simulink model "flight_controller"  (R2020a)
settings: Solver=FixedStepAuto  StartTime=0.0  StopTime=10  FixedStep=0.01  RelTol=1e-3
InitFcn:
  | flight_controller_setup % Run setup script for this simulation
values from neighbouring files (symbols this model uses):
  ki_dtheta = kp_dtheta*z_c    (= 0.1)    [PID_design_setup.m]
  kp_dtheta = 10^(K_dB/20)    [PID_design_setup.m]
  kp_theta = PID_theta.Kp    [flight_controller_setup.m]
  MM = [-1, 1 ... (first row only)    [flight_controller_payload_setup.m]    (also in flight_controller_setup.m)
  N_dtheta = Inf    (= inf)    [flight_controller_payload_setup.m]    (also in flight_controller_setup.m = 1/Tf_dtheta)
  N_dz = 5*2*pi    (= 31.4159265359)    [flight_controller_payload_setup.m]    (also in flight_controller_setup.m = 1/Tf_dz)
  x0 = zeros(nx,1)    [flight_controller_payload_setup.m]    (also in flight_controller_setup.m = zeros(6,1))
undefined symbols (not defined in the file or in its folder): kd_dtheta, kd_dz, ki_dz, kp_dz, kp_z
libraries: simulink x6
settings Model: Creator=murray  LastModifiedBy=murray

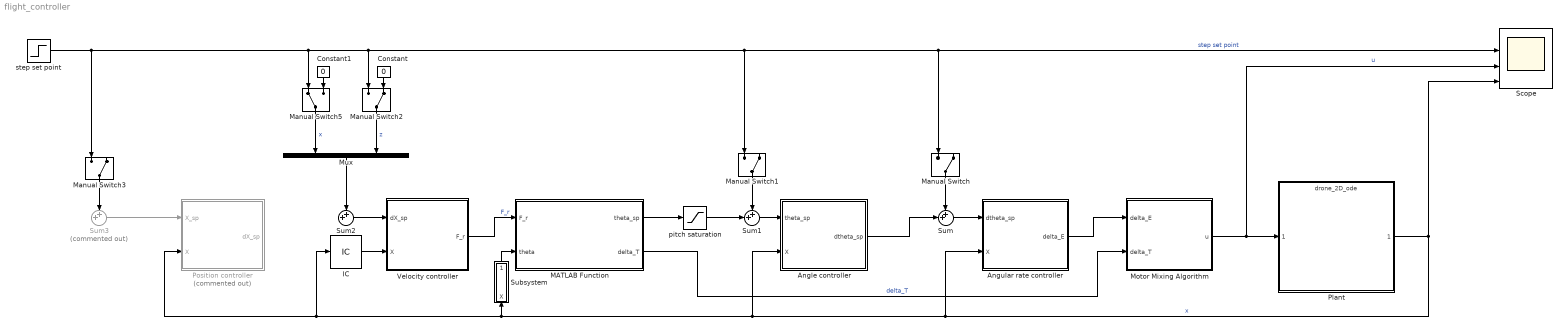
== system flight_controller ==
  Angle controller : Subsystem
  Angular rate controller : Subsystem
  Constant : Constant  Value=0
  Constant1 : Constant  Value=0
  IC : InitialCondition  Value=x0
  MATLAB Function : MATLAB Function  TreatAsAtomicUnit=on
  Manual Switch{,1..3} (4 alike) : ManualSwitch  CurrentSetting=0
  Manual Switch5 : ManualSwitch
  Motor Mixing Algorithm : Subsystem
  Mux : Mux  Inputs=2
  Plant : ModelReference  ModelNameDialog=drone_2D_ode  SimulationMode=Normal  ModelReferenceVersion=1.20
  Position controller : Subsystem  Commented=on
  Scope : Scope  NumInputPorts=4
  Subsystem : Subsystem
  Sum : Sum  Inputs=++|
  Sum1 : Sum  Inputs=++|
  Sum2 : Sum  Inputs=++|
  Sum3 : Sum  Commented=on  Inputs=++|
  Velocity controller : Subsystem
  pitch saturation : Saturate  UpperLimit=pi/2  LowerLimit=-pi/2
  step set point : Step  Time=2  SampleTime=0
  wires:
  Plant/1 -> Angle controller/2(X), IC/1, Position controller/2(X), Subsystem/1(X), Angular rate controller/2(X), Scope/4  "x"
  Angular rate controller/1(delta_E) -> Motor Mixing Algorithm/1(delta_E)
  MATLAB Function/2(delta_T) -> Motor Mixing Algorithm/2(delta_T)  "delta_T"
  Motor Mixing Algorithm/1(u) -> Scope/3, Plant/1  "u"
  Angle controller/1(dtheta_sp) -> Sum/2
  Sum/1 -> Angular rate controller/1(dtheta_sp)
  Manual Switch/1 -> Sum/1
  Manual Switch1/1 -> Sum1/1
  Sum1/1 -> Angle controller/1(theta_sp)
  step set point/1 -> Manual Switch/1, Scope/2, Manual Switch1/1, Manual Switch2/1, Manual Switch5/1, Manual Switch3/1  "step set point"
  Manual Switch3/1 -> Sum3/1
  Sum3/1 -> Position controller/1(X_sp)
  MATLAB Function/1(theta_sp) -> pitch saturation/1
  pitch saturation/1 -> Sum1/2
  Sum2/1 -> Velocity controller/1(dX_sp)
  Velocity controller/1(F_r) -> MATLAB Function/1(F_r)  "F_r"
  Manual Switch5/1 -> Mux/1  "x"
  Mux/1 -> Sum2/1
  IC/1 -> Velocity controller/2(X)
  Constant/1 -> Manual Switch2/2
  Constant1/1 -> Manual Switch5/2
  Manual Switch2/1 -> Mux/2  "z"
  Subsystem/1(theta) -> MATLAB Function/2(theta)

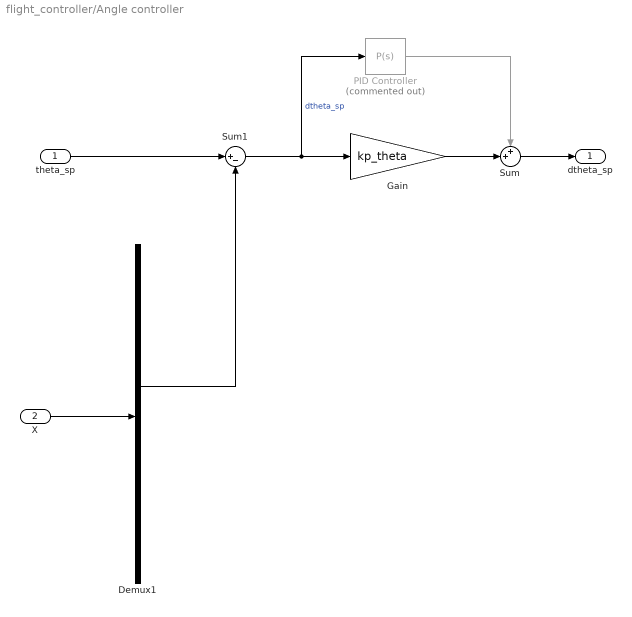
== system flight_controller/Angle controller ==
  theta_sp : Inport
  X : Inport  Port=2
  Demux1 : Demux  Outputs=6
  Gain : Gain  Gain=kp_theta
  PID Controller : simulink/Continuous/PID Controller  Commented=on  Controller=P  Form=Parallel  TimeDomain=Continuous-time  UseExternalTs=off  SampleTime=-1  IntegratorMethod=Forward Euler  FilterMethod=Forward Euler  ControllerParametersSource=internal  P=kp_theta  I=1  D=0  UseFilter=on  N=100  TunerSelectOption=Transfer Function Based (PID Tuner App)  InitialConditionSource=internal  InitialConditionForIntegrator=0  InitialConditionForFilter=0  DifferentiatorICPrevScaledInput=0  ExternalReset=none  TrackingMode=off  Kt=1  LimitOutput=off  UpperSaturationLimit=inf  LowerSaturationLimit=-inf  LinearizeAsGain=on  AntiWindupMode=none  Kb=1  POutMin=[]  POutMax=[]  IOutMin=[]  IOutMax=[]  DOutMin=[]  DOutMax=[]  NOutMin=[]  NOutMax=[]  SumOutMin=[]  SumOutMax=[]  SaturationOutMin=[]  SaturationOutMax=[]  PParamMin=[]  PParamMax=[]  IParamMin=[]  IParamMax=[]  DParamMin=[]  DParamMax=[]  NParamMin=[]  NParamMax=[]  KbParamMin=[]  KbParamMax=[]  KtParamMin=[]  KtParamMax=[]  KbOutMin=[]  KbOutMax=[]  KtOutMin=[]  KtOutMax=[]  IntegratorOutMin=[]  IntegratorOutMax=[]  FilterOutMin=[]  FilterOutMax=[]  SumI1OutMin=[]  SumI1OutMax=[]  SumI2OutMin=[]  SumI2OutMax=[]  SumI3OutMin=[]  SumI3OutMax=[]  SumI4OutMin=[]  SumI4OutMax=[]  SumDOutMin=[]  SumDOutMax=[]  DifferentiatorOutMin=[]  DifferentiatorOutMax=[]  FilterDiffOutCoefMin=[]  FilterDiffOutCoefMax=[]  ReciprocalOutMin=[]  ReciprocalOutMax=[]  SumDenOutMin=[]  SumDenOutMax=[]  SumNumOutMin=[]  SumNumOutMax=[]  DivideOutMin=[]  DivideOutMax=[]  UdiffTsProdOutMin=[]  UdiffTsProdOutMax=[]  NTsProdOutMin=[]  NTsProdOutMax=[]  UintegralTsProdOutMin=[]  UintegralTsProdOutMax=[]  UngainTsProdOutMin=[]  UngainTsProdOutMax=[]  IntegratorContinuousStateAttributes=''  IntegratorStateMustResolveToSignalObject=off  IntegratorRTWStateStorageClass=Auto  FilterContinuousStateAttributes=''  FilterStateMustResolveToSignalObject=off  FilterRTWStateStorageClass=Auto  ParallelPVariant=InternalParameters  IdealPVariant=Disabled  IVariant=Disabled  DVariant=Disabled  IntegratorVariant=Disabled  SatVariant=Disabled  AWVariant=Disabled  PCopyVariant=Disabled  TRVariant=Disabled  FdbkBlocksVariant=Forward  IdealPFdbkVariant=Disabled  SatFdbkVariant=Disabled  DerivativeFilterVariant=Disabled  NVariant=Disabled  NCopyVariant=Disabled_SignalSpec  FilterICVariant=Disabled  IntegratorICVariant=Disabled  ExternalResetVariant=Disabled  TRSumVariant=Passthrough  SumFdbkVariant=Disabled  SumVariant=Passthrough_P  TsampFilterVariant=InternalTs  TsampNgainVariant=Passthrough  TsampIntegralVariant=Disabled_SignalSpec
  Sum : Sum  Inputs=++|
  Sum1 : Sum  Inputs=|+-
  dtheta_sp : Outport
  wires:
  Sum1/1 -> PID Controller/1, Gain/1  "dtheta_sp"
  theta_sp/1 -> Sum1/1
  Sum/1 -> dtheta_sp/1
  PID Controller/1 -> Sum/1
  Gain/1 -> Sum/2
  X/1 -> Demux1/1
  Demux1/3 -> Sum1/2

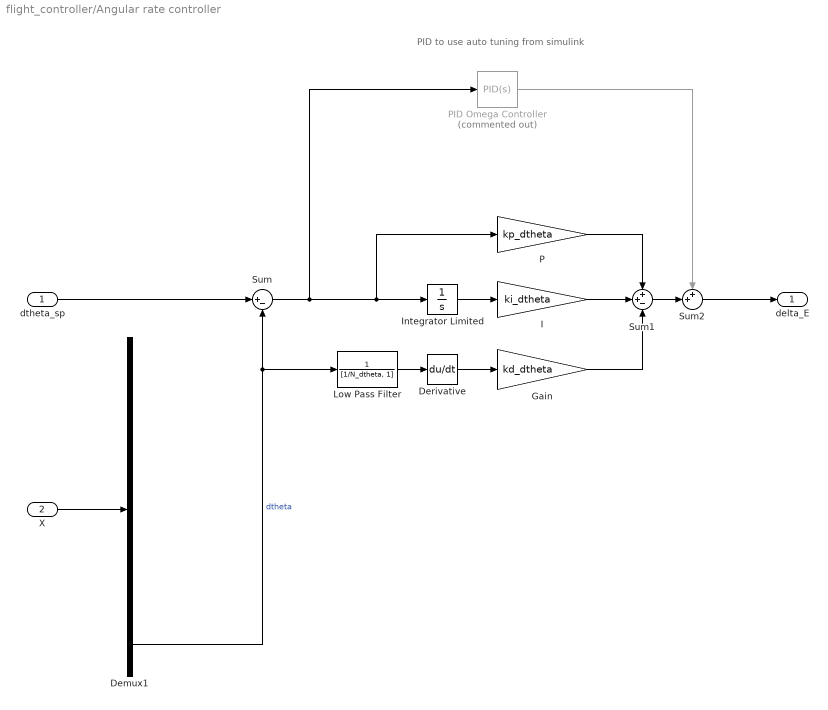
== system flight_controller/Angular rate controller ==
  note: PID to use auto tuning from simulink
  dtheta_sp : Inport
  X : Inport  Port=2
  Demux1 : Demux  Outputs=6
  Derivative : Derivative
  Gain : Gain  Gain=kd_dtheta
  I : Gain  Gain=ki_dtheta
  Integrator Limited : Integrator  LimitOutput=on  UpperSaturationLimit=10  LowerSaturationLimit=-10
  Low Pass Filter : TransferFcn  Denominator=[1/N_dtheta, 1]
  P : Gain  Gain=kp_dtheta
  PID Omega Controller : simulink/Continuous/PID Controller  Commented=on  Controller=PID  Form=Parallel  TimeDomain=Continuous-time  UseExternalTs=off  SampleTime=-1  IntegratorMethod=Forward Euler  FilterMethod=Forward Euler  ControllerParametersSource=internal  P=kp_dtheta  I=ki_dtheta  D=kd_dtheta  UseFilter=on  N=N_dtheta  TunerSelectOption=Transfer Function Based (PID Tuner App)  InitialConditionSource=internal  InitialConditionForIntegrator=0  InitialConditionForFilter=0  DifferentiatorICPrevScaledInput=0  ExternalReset=none  TrackingMode=off  Kt=1  LimitOutput=off  UpperSaturationLimit=inf  LowerSaturationLimit=-inf  LinearizeAsGain=on  AntiWindupMode=none  Kb=1  POutMin=[]  POutMax=[]  IOutMin=[]  IOutMax=[]  DOutMin=[]  DOutMax=[]  NOutMin=[]  NOutMax=[]  SumOutMin=[]  SumOutMax=[]  SaturationOutMin=[]  SaturationOutMax=[]  PParamMin=[]  PParamMax=[]  IParamMin=[]  IParamMax=[]  DParamMin=[]  DParamMax=[]  NParamMin=[]  NParamMax=[]  KbParamMin=[]  KbParamMax=[]  KtParamMin=[]  KtParamMax=[]  KbOutMin=[]  KbOutMax=[]  KtOutMin=[]  KtOutMax=[]  IntegratorOutMin=[]  IntegratorOutMax=[]  FilterOutMin=[]  FilterOutMax=[]  SumI1OutMin=[]  SumI1OutMax=[]  SumI2OutMin=[]  SumI2OutMax=[]  SumI3OutMin=[]  SumI3OutMax=[]  SumI4OutMin=[]  SumI4OutMax=[]  SumDOutMin=[]  SumDOutMax=[]  DifferentiatorOutMin=[]  DifferentiatorOutMax=[]  FilterDiffOutCoefMin=[]  FilterDiffOutCoefMax=[]  ReciprocalOutMin=[]  ReciprocalOutMax=[]  SumDenOutMin=[]  SumDenOutMax=[]  SumNumOutMin=[]  SumNumOutMax=[]  DivideOutMin=[]  DivideOutMax=[]  UdiffTsProdOutMin=[]  UdiffTsProdOutMax=[]  NTsProdOutMin=[]  NTsProdOutMax=[]  UintegralTsProdOutMin=[]  UintegralTsProdOutMax=[]  UngainTsProdOutMin=[]  UngainTsProdOutMax=[]  IntegratorContinuousStateAttributes=''  IntegratorStateMustResolveToSignalObject=off  IntegratorRTWStateStorageClass=Auto  FilterContinuousStateAttributes=''  FilterStateMustResolveToSignalObject=off  FilterRTWStateStorageClass=Auto  ParallelPVariant=InternalParameters  IdealPVariant=Disabled  IVariant=InternalParameters  DVariant=InternalParameters  IntegratorVariant=Continuous  SatVariant=Disabled  AWVariant=Passthrough  PCopyVariant=Disabled  TRVariant=Disabled  FdbkBlocksVariant=Forward  IdealPFdbkVariant=Disabled  SatFdbkVariant=Disabled  DerivativeFilterVariant=ContFilter  NVariant=InternalParameters  NCopyVariant=Disabled  FilterICVariant=InternalICsFilter  IntegratorICVariant=InternalICs  ExternalResetVariant=Disabled  TRSumVariant=Passthrough  SumFdbkVariant=Disabled  SumVariant=Sum_PID  TsampFilterVariant=InternalTs  TsampNgainVariant=Passthrough  TsampIntegralVariant=Passthrough
  Sum : Sum  Inputs=|+-
  Sum1 : Sum  Inputs=++-
  Sum2 : Sum  Inputs=++|
  delta_E : Outport
  wires:
  dtheta_sp/1 -> Sum/1
  Sum/1 -> P/1, Integrator Limited/1, PID Omega Controller/1
  Integrator Limited/1 -> I/1
  Derivative/1 -> Gain/1
  I/1 -> Sum1/2
  P/1 -> Sum1/1
  Gain/1 -> Sum1/3
  Sum1/1 -> Sum2/2
  Sum2/1 -> delta_E/1
  PID Omega Controller/1 -> Sum2/1
  Low Pass Filter/1 -> Derivative/1
  X/1 -> Demux1/1
  Demux1/6 -> Low Pass Filter/1, Sum/2  "dtheta"

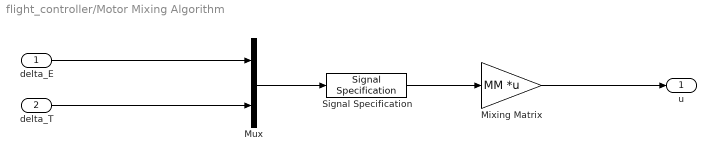
== system flight_controller/Motor Mixing Algorithm ==
  delta_E : Inport
  delta_T : Inport  Port=2
  Mixing Matrix : Gain  Gain=MM  Multiplication=Matrix(K*u)
  Mux : Mux  Inputs=2
  Signal Specification : SignalSpecification  Dimensions=[2, 1]
  u : Outport  LockScale=on
  wires:
  delta_T/1 -> Mux/2
  delta_E/1 -> Mux/1
  Mixing Matrix/1 -> u/1
  Mux/1 -> Signal Specification/1
  Signal Specification/1 -> Mixing Matrix/1

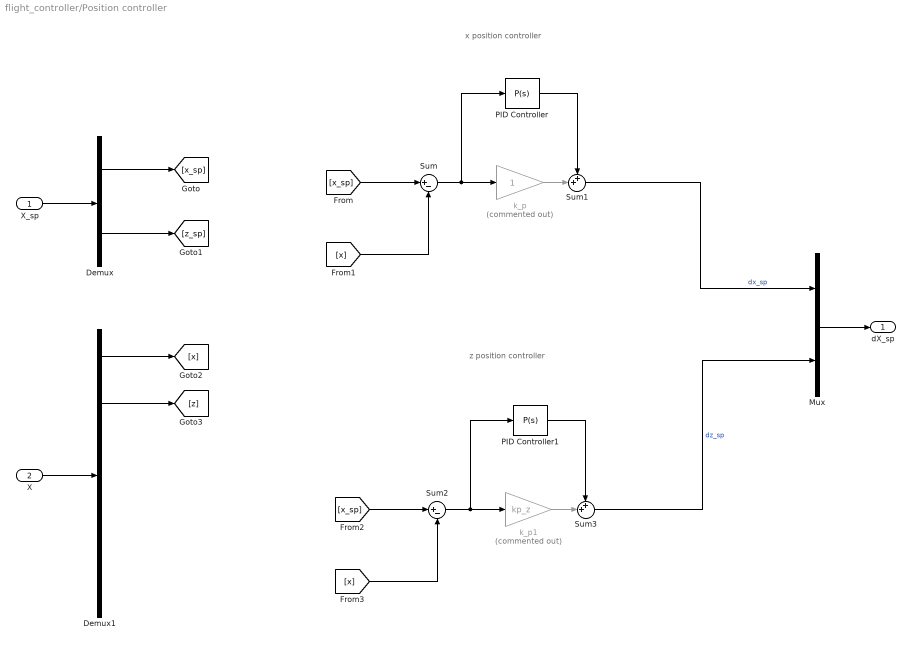
== system flight_controller/Position controller ==
  note: x position controller
  note: z position controller
  X_sp : Inport
  X : Inport  Port=2
  Demux : Demux  Outputs=2
  Demux1 : Demux  Outputs=6
  Mux : Mux  Inputs=2
  PID Controller : simulink/Continuous/PID Controller  Controller=P  Form=Parallel  TimeDomain=Continuous-time  UseExternalTs=off  SampleTime=-1  IntegratorMethod=Forward Euler  FilterMethod=Forward Euler  ControllerParametersSource=internal  P=1  I=1  D=0  UseFilter=on  N=100  TunerSelectOption=Transfer Function Based (PID Tuner App)  InitialConditionSource=internal  InitialConditionForIntegrator=0  InitialConditionForFilter=0  DifferentiatorICPrevScaledInput=0  ExternalReset=none  TrackingMode=off  Kt=1  LimitOutput=off  UpperSaturationLimit=inf  LowerSaturationLimit=-inf  LinearizeAsGain=on  AntiWindupMode=none  Kb=1  POutMin=[]  POutMax=[]  IOutMin=[]  IOutMax=[]  DOutMin=[]  DOutMax=[]  NOutMin=[]  NOutMax=[]  SumOutMin=[]  SumOutMax=[]  SaturationOutMin=[]  SaturationOutMax=[]  PParamMin=[]  PParamMax=[]  IParamMin=[]  IParamMax=[]  DParamMin=[]  DParamMax=[]  NParamMin=[]  NParamMax=[]  KbParamMin=[]  KbParamMax=[]  KtParamMin=[]  KtParamMax=[]  KbOutMin=[]  KbOutMax=[]  KtOutMin=[]  KtOutMax=[]  IntegratorOutMin=[]  IntegratorOutMax=[]  FilterOutMin=[]  FilterOutMax=[]  SumI1OutMin=[]  SumI1OutMax=[]  SumI2OutMin=[]  SumI2OutMax=[]  SumI3OutMin=[]  SumI3OutMax=[]  SumI4OutMin=[]  SumI4OutMax=[]  SumDOutMin=[]  SumDOutMax=[]  DifferentiatorOutMin=[]  DifferentiatorOutMax=[]  FilterDiffOutCoefMin=[]  FilterDiffOutCoefMax=[]  ReciprocalOutMin=[]  ReciprocalOutMax=[]  SumDenOutMin=[]  SumDenOutMax=[]  SumNumOutMin=[]  SumNumOutMax=[]  DivideOutMin=[]  DivideOutMax=[]  UdiffTsProdOutMin=[]  UdiffTsProdOutMax=[]  NTsProdOutMin=[]  NTsProdOutMax=[]  UintegralTsProdOutMin=[]  UintegralTsProdOutMax=[]  UngainTsProdOutMin=[]  UngainTsProdOutMax=[]  IntegratorContinuousStateAttributes=''  IntegratorStateMustResolveToSignalObject=off  IntegratorRTWStateStorageClass=Auto  FilterContinuousStateAttributes=''  FilterStateMustResolveToSignalObject=off  FilterRTWStateStorageClass=Auto  ParallelPVariant=InternalParameters  IdealPVariant=Disabled  IVariant=Disabled  DVariant=Disabled  IntegratorVariant=Disabled  SatVariant=Disabled  AWVariant=Disabled  PCopyVariant=Disabled  TRVariant=Disabled  FdbkBlocksVariant=Forward  IdealPFdbkVariant=Disabled  SatFdbkVariant=Disabled  DerivativeFilterVariant=Disabled  NVariant=Disabled  NCopyVariant=Disabled_SignalSpec  FilterICVariant=Disabled  IntegratorICVariant=Disabled  ExternalResetVariant=Disabled  TRSumVariant=Passthrough  SumFdbkVariant=Disabled  SumVariant=Passthrough_P  TsampFilterVariant=InternalTs  TsampNgainVariant=Passthrough  TsampIntegralVariant=Disabled_SignalSpec
  PID Controller1 : simulink/Continuous/PID Controller  Controller=P  Form=Parallel  TimeDomain=Continuous-time  UseExternalTs=off  SampleTime=-1  IntegratorMethod=Forward Euler  FilterMethod=Forward Euler  ControllerParametersSource=internal  P=kp_z  I=1  D=0  UseFilter=on  N=100  TunerSelectOption=Transfer Function Based (PID Tuner App)  InitialConditionSource=internal  InitialConditionForIntegrator=0  InitialConditionForFilter=0  DifferentiatorICPrevScaledInput=0  ExternalReset=none  TrackingMode=off  Kt=1  LimitOutput=off  UpperSaturationLimit=inf  LowerSaturationLimit=-inf  LinearizeAsGain=on  AntiWindupMode=none  Kb=1  POutMin=[]  POutMax=[]  IOutMin=[]  IOutMax=[]  DOutMin=[]  DOutMax=[]  NOutMin=[]  NOutMax=[]  SumOutMin=[]  SumOutMax=[]  SaturationOutMin=[]  SaturationOutMax=[]  PParamMin=[]  PParamMax=[]  IParamMin=[]  IParamMax=[]  DParamMin=[]  DParamMax=[]  NParamMin=[]  NParamMax=[]  KbParamMin=[]  KbParamMax=[]  KtParamMin=[]  KtParamMax=[]  KbOutMin=[]  KbOutMax=[]  KtOutMin=[]  KtOutMax=[]  IntegratorOutMin=[]  IntegratorOutMax=[]  FilterOutMin=[]  FilterOutMax=[]  SumI1OutMin=[]  SumI1OutMax=[]  SumI2OutMin=[]  SumI2OutMax=[]  SumI3OutMin=[]  SumI3OutMax=[]  SumI4OutMin=[]  SumI4OutMax=[]  SumDOutMin=[]  SumDOutMax=[]  DifferentiatorOutMin=[]  DifferentiatorOutMax=[]  FilterDiffOutCoefMin=[]  FilterDiffOutCoefMax=[]  ReciprocalOutMin=[]  ReciprocalOutMax=[]  SumDenOutMin=[]  SumDenOutMax=[]  SumNumOutMin=[]  SumNumOutMax=[]  DivideOutMin=[]  DivideOutMax=[]  UdiffTsProdOutMin=[]  UdiffTsProdOutMax=[]  NTsProdOutMin=[]  NTsProdOutMax=[]  UintegralTsProdOutMin=[]  UintegralTsProdOutMax=[]  UngainTsProdOutMin=[]  UngainTsProdOutMax=[]  IntegratorContinuousStateAttributes=''  IntegratorStateMustResolveToSignalObject=off  IntegratorRTWStateStorageClass=Auto  FilterContinuousStateAttributes=''  FilterStateMustResolveToSignalObject=off  FilterRTWStateStorageClass=Auto  ParallelPVariant=InternalParameters  IdealPVariant=Disabled  IVariant=Disabled  DVariant=Disabled  IntegratorVariant=Disabled  SatVariant=Disabled  AWVariant=Disabled  PCopyVariant=Disabled  TRVariant=Disabled  FdbkBlocksVariant=Forward  IdealPFdbkVariant=Disabled  SatFdbkVariant=Disabled  DerivativeFilterVariant=Disabled  NVariant=Disabled  NCopyVariant=Disabled_SignalSpec  FilterICVariant=Disabled  IntegratorICVariant=Disabled  ExternalResetVariant=Disabled  TRSumVariant=Passthrough  SumFdbkVariant=Disabled  SumVariant=Passthrough_P  TsampFilterVariant=InternalTs  TsampNgainVariant=Passthrough  TsampIntegralVariant=Disabled_SignalSpec
  Sum : Sum  Inputs=|+-
  Sum1 : Sum  Inputs=++|
  Sum2 : Sum  Inputs=|+-
  Sum3 : Sum  Inputs=++|
  k_p : Gain  Commented=on
  k_p1 : Gain  Commented=on  Gain=kp_z
  dX_sp : Outport
  wires:
  Sum/1 -> PID Controller/1, k_p/1
  k_p/1 -> Sum1/2
  PID Controller/1 -> Sum1/1
  X_sp/1 -> Demux/1
  Demux/2 -> [z_sp]
  Demux/1 -> [x_sp]
  X/1 -> Demux1/1
  Demux1/1 -> [x]
  Demux1/2 -> [z]
  [x_sp] -> Sum/1
  [x] -> Sum/2
  Sum2/1 -> PID Controller1/1, k_p1/1
  [x] -> Sum2/2
  [x_sp] -> Sum2/1
  PID Controller1/1 -> Sum3/1
  Sum3/1 -> Mux/2  "dz_sp"
  k_p1/1 -> Sum3/2
  Mux/1 -> dX_sp/1
  Sum1/1 -> Mux/1  "dx_sp"

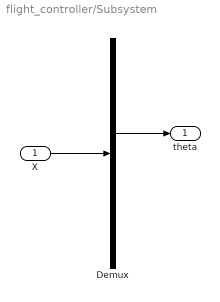
== system flight_controller/Subsystem ==
  X : Inport
  Demux : Demux  Outputs=6
  theta : Outport
  wires:
  X/1 -> Demux/1
  Demux/3 -> theta/1

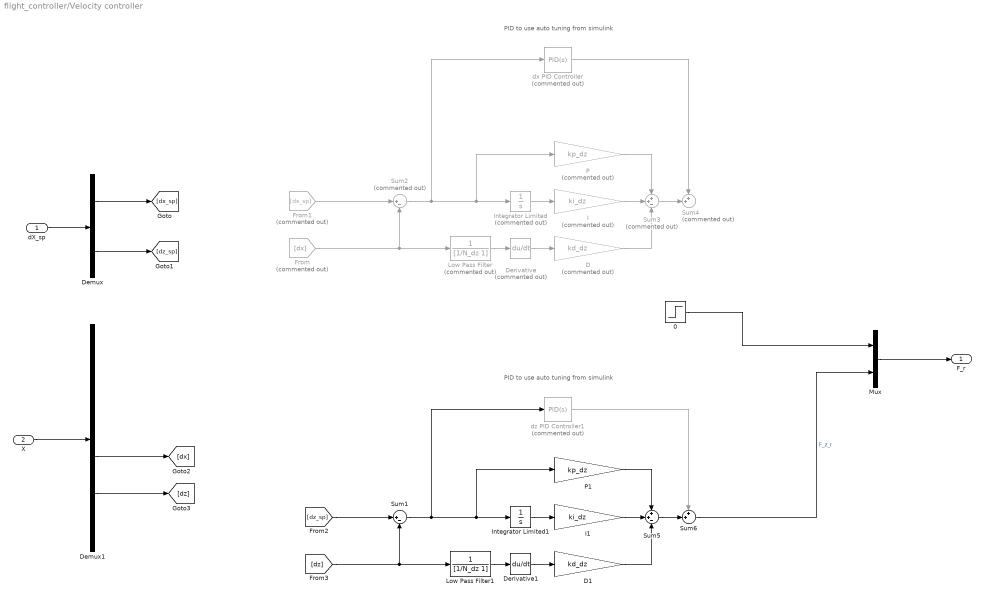
== system flight_controller/Velocity controller ==
  note: PID to use auto tuning from simulink
  note: PID to use auto tuning from simulink
  dX_sp : Inport
  X : Inport  Port=2
  0 : Step  After=0  SampleTime=0
  D : Gain  Commented=on  Gain=kd_dz
  D1 : Gain  Gain=kd_dz
  Demux : Demux  Outputs=2
  Demux1 : Demux  Outputs=6
  Derivative : Derivative  Commented=on
  Derivative1 : Derivative
  From : From  Commented=on  GotoTag=dx
  From1 : From  Commented=on  GotoTag=dx_sp
  I : Gain  Commented=on  Gain=ki_dz
  I1 : Gain  Gain=ki_dz
  Integrator Limited : Integrator  Commented=on  LimitOutput=on  UpperSaturationLimit=10  LowerSaturationLimit=-10
  Integrator Limited1 : Integrator  LimitOutput=on  UpperSaturationLimit=10  LowerSaturationLimit=-10
  Low Pass Filter : TransferFcn  Commented=on  Denominator=[1/N_dz 1]
  Low Pass Filter1 : TransferFcn  Denominator=[1/N_dz 1]
  Mux : Mux  Inputs=2
  P : Gain  Commented=on  Gain=kp_dz
  P1 : Gain  Gain=kp_dz
  Sum1 : Sum  Inputs=|+-
  Sum2 : Sum  Commented=on  Inputs=|+-
  Sum3 : Sum  Commented=on  Inputs=++-
  Sum4 : Sum  Commented=on  Inputs=++|
  Sum5 : Sum  Inputs=++-
  Sum6 : Sum  Inputs=++|
  dx PID Controller : simulink/Continuous/PID Controller  Commented=on  Controller=PID  Form=Parallel  TimeDomain=Continuous-time  UseExternalTs=off  SampleTime=-1  IntegratorMethod=Forward Euler  FilterMethod=Forward Euler  ControllerParametersSource=internal  P=1  I=1  D=0  UseFilter=on  N=10  TunerSelectOption=Transfer Function Based (PID Tuner App)  InitialConditionSource=internal  InitialConditionForIntegrator=0  InitialConditionForFilter=0  DifferentiatorICPrevScaledInput=0  ExternalReset=none  TrackingMode=off  Kt=1  LimitOutput=off  UpperSaturationLimit=inf  LowerSaturationLimit=-inf  LinearizeAsGain=on  AntiWindupMode=none  Kb=1  POutMin=[]  POutMax=[]  IOutMin=[]  IOutMax=[]  DOutMin=[]  DOutMax=[]  NOutMin=[]  NOutMax=[]  SumOutMin=[]  SumOutMax=[]  SaturationOutMin=[]  SaturationOutMax=[]  PParamMin=[]  PParamMax=[]  IParamMin=[]  IParamMax=[]  DParamMin=[]  DParamMax=[]  NParamMin=[]  NParamMax=[]  KbParamMin=[]  KbParamMax=[]  KtParamMin=[]  KtParamMax=[]  KbOutMin=[]  KbOutMax=[]  KtOutMin=[]  KtOutMax=[]  IntegratorOutMin=[]  IntegratorOutMax=[]  FilterOutMin=[]  FilterOutMax=[]  SumI1OutMin=[]  SumI1OutMax=[]  SumI2OutMin=[]  SumI2OutMax=[]  SumI3OutMin=[]  SumI3OutMax=[]  SumI4OutMin=[]  SumI4OutMax=[]  SumDOutMin=[]  SumDOutMax=[]  DifferentiatorOutMin=[]  DifferentiatorOutMax=[]  FilterDiffOutCoefMin=[]  FilterDiffOutCoefMax=[]  ReciprocalOutMin=[]  ReciprocalOutMax=[]  SumDenOutMin=[]  SumDenOutMax=[]  SumNumOutMin=[]  SumNumOutMax=[]  DivideOutMin=[]  DivideOutMax=[]  UdiffTsProdOutMin=[]  UdiffTsProdOutMax=[]  NTsProdOutMin=[]  NTsProdOutMax=[]  UintegralTsProdOutMin=[]  UintegralTsProdOutMax=[]  UngainTsProdOutMin=[]  UngainTsProdOutMax=[]  IntegratorContinuousStateAttributes=''  IntegratorStateMustResolveToSignalObject=off  IntegratorRTWStateStorageClass=Auto  FilterContinuousStateAttributes=''  FilterStateMustResolveToSignalObject=off  FilterRTWStateStorageClass=Auto  ParallelPVariant=InternalParameters  IdealPVariant=Disabled  IVariant=InternalParameters  DVariant=InternalParameters  IntegratorVariant=Continuous  SatVariant=Disabled  AWVariant=Passthrough  PCopyVariant=Disabled  TRVariant=Disabled  FdbkBlocksVariant=Forward  IdealPFdbkVariant=Disabled  SatFdbkVariant=Disabled  DerivativeFilterVariant=ContFilter  NVariant=InternalParameters  NCopyVariant=Disabled  FilterICVariant=InternalICsFilter  IntegratorICVariant=InternalICs  ExternalResetVariant=Disabled  TRSumVariant=Passthrough  SumFdbkVariant=Disabled  SumVariant=Sum_PID  TsampFilterVariant=InternalTs  TsampNgainVariant=Passthrough  TsampIntegralVariant=Passthrough
  dz PID Controller1 : simulink/Continuous/PID Controller  Commented=on  Controller=PID  Form=Parallel  TimeDomain=Continuous-time  UseExternalTs=off  SampleTime=-1  IntegratorMethod=Forward Euler  FilterMethod=Forward Euler  ControllerParametersSource=internal  P=kp_dz  I=ki_dz  D=kd_dz  UseFilter=on  N=N_dz  TunerSelectOption=Transfer Function Based (PID Tuner App)  InitialConditionSource=internal  InitialConditionForIntegrator=0  InitialConditionForFilter=0  DifferentiatorICPrevScaledInput=0  ExternalReset=none  TrackingMode=off  Kt=1  LimitOutput=off  UpperSaturationLimit=inf  LowerSaturationLimit=-inf  LinearizeAsGain=on  AntiWindupMode=none  Kb=1  POutMin=[]  POutMax=[]  IOutMin=[]  IOutMax=[]  DOutMin=[]  DOutMax=[]  NOutMin=[]  NOutMax=[]  SumOutMin=[]  SumOutMax=[]  SaturationOutMin=[]  SaturationOutMax=[]  PParamMin=[]  PParamMax=[]  IParamMin=[]  IParamMax=[]  DParamMin=[]  DParamMax=[]  NParamMin=[]  NParamMax=[]  KbParamMin=[]  KbParamMax=[]  KtParamMin=[]  KtParamMax=[]  KbOutMin=[]  KbOutMax=[]  KtOutMin=[]  KtOutMax=[]  IntegratorOutMin=[]  IntegratorOutMax=[]  FilterOutMin=[]  FilterOutMax=[]  SumI1OutMin=[]  SumI1OutMax=[]  SumI2OutMin=[]  SumI2OutMax=[]  SumI3OutMin=[]  SumI3OutMax=[]  SumI4OutMin=[]  SumI4OutMax=[]  SumDOutMin=[]  SumDOutMax=[]  DifferentiatorOutMin=[]  DifferentiatorOutMax=[]  FilterDiffOutCoefMin=[]  FilterDiffOutCoefMax=[]  ReciprocalOutMin=[]  ReciprocalOutMax=[]  SumDenOutMin=[]  SumDenOutMax=[]  SumNumOutMin=[]  SumNumOutMax=[]  DivideOutMin=[]  DivideOutMax=[]  UdiffTsProdOutMin=[]  UdiffTsProdOutMax=[]  NTsProdOutMin=[]  NTsProdOutMax=[]  UintegralTsProdOutMin=[]  UintegralTsProdOutMax=[]  UngainTsProdOutMin=[]  UngainTsProdOutMax=[]  IntegratorContinuousStateAttributes=''  IntegratorStateMustResolveToSignalObject=off  IntegratorRTWStateStorageClass=Auto  FilterContinuousStateAttributes=''  FilterStateMustResolveToSignalObject=off  FilterRTWStateStorageClass=Auto  ParallelPVariant=InternalParameters  IdealPVariant=Disabled  IVariant=InternalParameters  DVariant=InternalParameters  IntegratorVariant=Continuous  SatVariant=Disabled  AWVariant=Passthrough  PCopyVariant=Disabled  TRVariant=Disabled  FdbkBlocksVariant=Forward  IdealPFdbkVariant=Disabled  SatFdbkVariant=Disabled  DerivativeFilterVariant=ContFilter  NVariant=InternalParameters  NCopyVariant=Disabled  FilterICVariant=InternalICsFilter  IntegratorICVariant=InternalICs  ExternalResetVariant=Disabled  TRSumVariant=Passthrough  SumFdbkVariant=Disabled  SumVariant=Sum_PID  TsampFilterVariant=InternalTs  TsampNgainVariant=Passthrough  TsampIntegralVariant=Passthrough
  F_r : Outport
  wires:
  Derivative/1 -> D/1
  Sum3/1 -> Sum4/2
  Sum2/1 -> dx PID Controller/1, P/1, Integrator Limited/1
  I/1 -> Sum3/2
  Integrator Limited/1 -> I/1
  dx PID Controller/1 -> Sum4/1
  P/1 -> Sum3/1
  Low Pass Filter/1 -> Derivative/1
  D/1 -> Sum3/3
  Mux/1 -> F_r/1
  P1/1 -> Sum5/1
  Integrator Limited1/1 -> I1/1
  dz PID Controller1/1 -> Sum6/1
  I1/1 -> Sum5/2
  Sum1/1 -> dz PID Controller1/1, P1/1, Integrator Limited1/1
  Sum5/1 -> Sum6/2
  Low Pass Filter1/1 -> Derivative1/1
  Derivative1/1 -> D1/1
  D1/1 -> Sum5/3
  dX_sp/1 -> Demux/1
  X/1 -> Demux1/1
  From/1 -> Sum2/2, Low Pass Filter/1
  From1/1 -> Sum2/1
  Demux/1 -> [dx_sp]
  Demux/2 -> [dz_sp]
  [dz] -> Sum1/2, Low Pass Filter1/1
  [dz_sp] -> Sum1/1
  Demux1/4 -> [dx]
  Demux1/5 -> [dz]
  0/1 -> Mux/1
  Sum6/1 -> Mux/2  "F_z_r"

== matlab function flight_controller/MATLAB Function ==
  data: F_r input; theta_sp output; delta_T output; theta input
function [theta_sp, delta_T]= inertial_to_body(F_r, theta)
%% Converts forces in inertial frame to body references (thrust and pitch reference)
% theta_sp = pitch set point
% delta_T = thrust reference
% F_r = [F_x_r, F_y_r], reference force vector in inertial frame

% NB: z is positive in down direction

delta_T = -F_r(2)/cos(theta);

theta_sp = -asin(min(max((F_r(1)/delta_T),-1),1)); % arcsine of bounded fraction. magnitude not larger than 1

end
